simulink model "HarnessModel_MotorDrive"  (R2025a)
settings: Solver=VariableStepAuto  StartTime=0.0  StopTime=0.2  MaxStep=1/2e-6  RelTol=1e-3  AbsTol=1e-3  EnableMultiTasking=on
PreLoadFcn:
  | HarnessSetup_MotorDrive
undefined symbols (not defined in the file or in its folder): foc, PmsmFem, testParams
libraries: nesl_utility x14, ee_lib x12, fl_lib x10, spsFirstOrderFilterLib x4, eePmsmFieldOrientedControl x1
(part 1 of 2)
Description:
  | Three-Phase PMSM Drive
settings Model: Creator=The MathWorks, Inc.  LastModifiedBy=isaacito
settings SolverCC: AutoScaleAbsTol=off  MaxConsecutiveMinStep=2  ZeroCrossAlgorithm=Adaptive  AlgebraicLoopSolver=TrustRegion
settings DataIOCC: LimitDataPoints=on  MaxDataPoints=690000  SaveFormat=Array  InspectSignalLogs=on
settings OptimizationCC: LifeSpan=inf
settings DebuggingCC: UnderspecifiedInitializationDetection=Classic  MergeDetectMultiDrivingBlocksExec=none  MaxConsecutiveZCsMsg=none  IgnoredZcDiagnostic=none  UnconnectedInputMsg=warning  UnconnectedOutputMsg=warning  UnconnectedLineMsg=warning  AllowSymbolicDim=off  PregeneratedLibrarySubsystemCodeDiagnostic=none  SFUnexpectedBacktrackingDiag=warning  SFNoUnconditionalDefaultTransitionDiag=warning  SFExecutionAtInitializationDiag=none  ArithmeticOperatorsInVariantConditions=warning
settings HardwareCC: ProdBitPerPointer=32.0  ProdBitPerSizeT=32.0  ProdBitPerPtrDiffT=32.0  ProdLargestAtomicFloat=None  ProdIntDivRoundTo=Undefined  ProdEndianess=Unspecified  ProdWordSize=32.0  ProdHWDeviceType=32-bit Generic
settings ModelReferenceCC: EnableRefExpFcnMdlSchedulingChecks=on  PropagateSignalLabelsOutOfModel=off
settings SFSimCC: SimUseLocalCustomCode=off  CustomCodeUndefinedFunction=UseInterfaceOnly
settings RTWCC: RTWUseLocalCustomCode=off  GPUComputeCapability=3.5
settings CodeAppCC: StateflowObjectComments=on
settings GRTTargetCC: TargetLangStandard=C89/C90 (ANSI)
settings ConfigComp: CovMetricSettings=dw  CovSaveCumulativeToWorkspaceVar=on  CovSaveSingleToWorkspaceVar=on  CovExternalEMLEnable=off  CovSFcnEnable=off
settings SimscapeCC: SimscapeLogType=local  SimscapeLogName=logsoutssc  SimscapeLogLimitData=off  SimscapeLogDataHistory=1000000.0

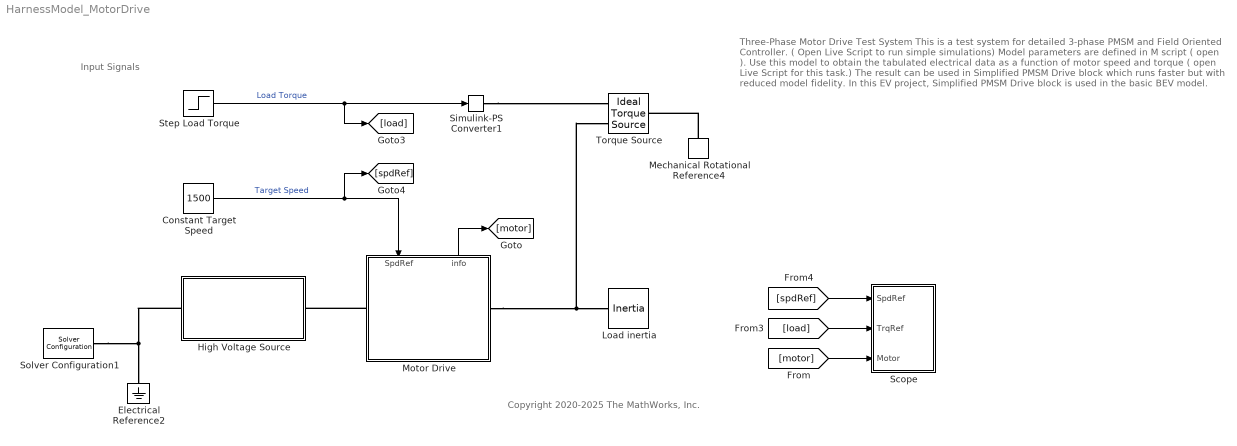
== system HarnessModel_MotorDrive ==
  note: Copyright 2020-2025 The MathWorks, Inc.
  note: Input Signals
  note: Three-Phase Motor Drive Test System
      |
      | This is a test system for detailed 3-phase PMSM and Field Oriented
      | Controller. ( Open Live Script to run simple simulations)
      |
      | Model parameters are defined in M script ( open ).
      |
      | Use this model to obtain the tabulated electrical data as a function of
      | motor speed and torque ( open Live Script for this task.) The result can be
      | used in Simplified PMSM Drive block which runs faster but with reduced
      | model fidelity. In this EV project, Simplified PMSM Drive block is used in
      | the basic BEV model.
  Constant Target Speed : Constant  Value=1500  SampleTime=testParams.controlSampleTime_s
      settings: AttributesFormatString=%<SampleTime>
  Electrical Reference2 : fl_lib/Electrical/Electrical Elements/Electrical Reference
  High Voltage Source : Subsystem
  Load inertia : fl_lib/Mechanical/Rotational Elements/Inertia  inertia=testParams.Load_Inertia_kg_m2 kg*m^2  num_ports=foundation.enum.numPorts2.one  w_specify=on  w_priority=High  w=1500 rpm  w_nominal_specify=off  w_nominal_value=1  w_nominal_unit=rad/s  t_specify=off  t_priority=High  t=0 N*m  t_nominal_specify=off  t_nominal_value=1  t_nominal_unit=N*m
      settings: AttributesFormatString=Initial %<w> %<w_unit>
  Mechanical Rotational Reference4 : fl_lib/Mechanical/Rotational Elements/Mechanical Rotational Reference
  Motor Drive : Subsystem
      settings: PortSchema="{\"entries\":[{\"content\":{\"sides\":[{\"content\":{\"connectorIds\":[\"LConn1\"]},\"type\":\"ConnectorPlacement.EquallySpacedRectSide\",\"uuid\":\"01e463d5-292f-49ad-b53f-26bdaef9861a\"},{\"content\":{\"connectorIds\":[\"RConn1\"],\"side\":\"RIGHT\"},\"type\":\"ConnectorPlacement.EquallySpacedRectSide\",\"uuid\":\"c82e9c8b-ca5a-45cd-a1e1-09f3eb3693bb\"},{\"content\":{\"connectorIds\":[\"In1\",\"Out1\"],\"side\":\"TOP\"},\"type\":\"ConnectorPlacement.EquallySpacedRectSide\",\"uuid\":\"d9b13513-5e9a-4a5c-9a36-dd7bb14f7238\"}]},\"type\":\"ConnectorPlacement.EquallySpacedConnector\",\"uuid\":\"1701c5a8-0236-4c04-8589-5cbcf2c3bfdc\"}],\"packageUris\":[\"http://schema.mathworks.com/mf0/Connector/19700101\"],\"version\":\"1.0\"}"
  Scope : Subsystem
  Simulink-PS Converter1 : nesl_utility/Simulink-PS Converter  PhysicalDomain=network_engine_domain  SubClassName=ps_input  LeftPortType=input  RightPortType=output  PseudoPeriodic=off  Frequencies=[]  NoiseDistribution=none  NoiseParameters=[]  Unit=N*m  AffineConversion=off  FilteringAndDerivatives=provide  SimscapeFilterOrder=1  InputFilterTimeConstant=0.001  UdotUserProvided=0
  Solver Configuration1 : nesl_utility/Solver Configuration  PhysicalDomain=network_engine_domain  SubClassName=solver  LeftPortType=input  RightPortType=generic  Tones=[]  Harmonics=[]  SimulateNoise=off  Profile=off  UseLocalSampling=off  EnableSwitchedLinearOptims=on  FrequencyDomain=off  UseCCode=off  RelTol=0.001  AbsTol=1e-06  MinStep=1e-09  ToWorkspace=off  RevertToSquareIcSolve=off  NumHomotopyIterations=100  PhasorMode=off  PhasorModeNumHarmonics=1  ConsistencySolver=NEWTON_FTOL  IndexReductionMethod=DerivativeReplacement  DoDC=off  ResidualTolerance=1e-9  ConsistencyTolSource=GLOBAL  ConsistencyAbsTol=0.001  ConsistencyRelTol=0.001  ConsistencyTolFactor=0.001  UseLocalSolver=on  LocalSolverChoice=NE_BACKWARD_EULER_ADVANCER  ResolveIndetEquations=on  FunctionEvalNumThread=1  LocalSolverSampleTime=testParams.sampleTime_s  DoFixedCost=on  MaxNonlinIter=5  MaxModeIter=2  ComputeImpulses=off  ImpulseIterations=2  LinearAlgebra=auto  LinearAlgebraNumThread=0  EquationFormulation=NE_TIME_EF  DelaysMemoryBudget=1024  AutomaticFiltering=on  FilteringTimeConstant=0.001  PartitionStorageMethod=AS_NEEDED  PartitionMemoryBudget=1024  PartitionMethod=FAST  MultibodyUseLocalSolver=off  MultibodyLocalSolverChoice=ODE1  MultibodyLocalSolverSampleTime=0.001
      settings: AttributesFormatString=Local solver %<UseLocalSolver>
  Step Load Torque : Step  Time=0.01  After=150  SampleTime=0
      settings: AttributesFormatString=|
      | Initial %<Before>
      | Step to %<After>
  Torque Source : fl_lib/Mechanical/Mechanical Sources/Ideal Torque Source
  wires:
  Step Load Torque/1 -> [load], Simulink-PS Converter1/1  "Load Torque"
  Motor Drive/1(info) -> [motor]
  Constant Target Speed/1 -> [spdRef], Motor Drive/1(SpdRef)  "Target Speed"
  [spdRef] -> Scope/1(SpdRef)
  [load] -> Scope/2(TrqRef)
  [motor] -> Scope/3(Motor)
  connections:
  Motor Drive/RConn1 -- Torque Source/RConn2 -- Load inertia/LConn1
  Simulink-PS Converter1/RConn1 -- Torque Source/RConn1
  Mechanical Rotational Reference4/LConn1 -- Torque Source/LConn1
  Motor Drive/LConn1 -- High Voltage Source/RConn1
  High Voltage Source/LConn1 -- Electrical Reference2/LConn1 -- Solver Configuration1/RConn1

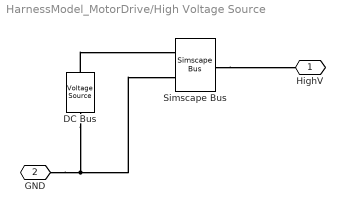
== system HarnessModel_MotorDrive/High Voltage Source ==
  DC Bus : ee_lib/Sources/Voltage Source  dc_voltage=testParams.DC_V V  ac_voltage=0 V  ac_shift=0 deg  ac_frequency=0 Hz  noise_mode=0  PSD=0 V^2/Hz  sample_time=0.001 s  repeatability=1  user_seed=0  auto_seed=2280074224  i_specify=off  i_priority=None  i=0 A  i_nominal_specify=off  i_nominal_value=1  i_nominal_unit=A  v_specify=off  v_priority=None  v=0 V  v_nominal_specify=off  v_nominal_value=1  v_nominal_unit=V
      settings: AttributesFormatString=%<dc_voltage> (%<dc_voltage_unit>)
  Simscape Bus : SimscapeBus  HierarchyStrings=plus;minus
  HighV : PMIOPort  Side=Right
  GND : PMIOPort  Port=2  Side=Left
  connections:
  DC Bus/LConn1 -- Simscape Bus/LConn1
  DC Bus/RConn1 -- GND/RConn1 -- Simscape Bus/LConn2
  Simscape Bus/RConn1 -- HighV/RConn1

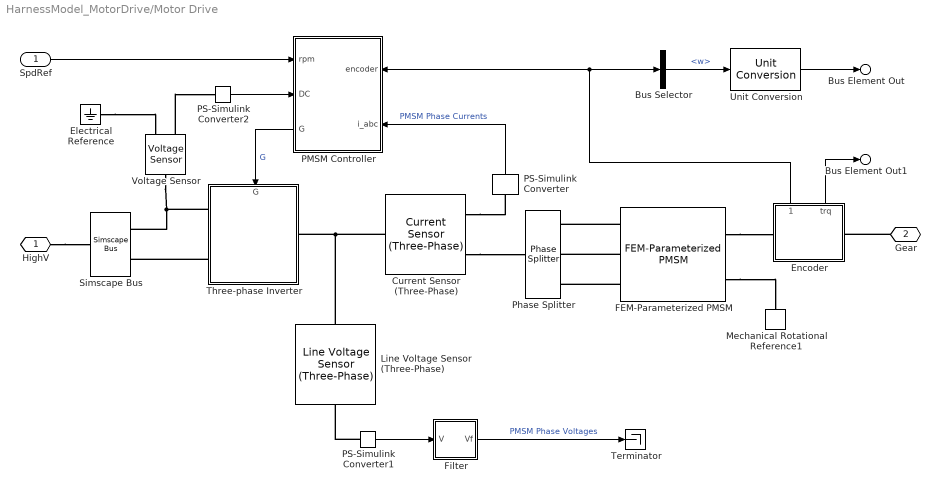
== system HarnessModel_MotorDrive/Motor Drive ==
  SpdRef : Inport  Unit=rpm
  Bus Selector : BusSelector  OutputSignals=w
  Current Sensor (Three-Phase) : ee_lib/Sensors & Transducers/Current Sensor (Three-Phase)
  Electrical Reference : fl_lib/Electrical/Electrical Elements/Electrical Reference
  Encoder : Subsystem
      settings: PortSchema="{\"entries\":[{\"content\":{\"sides\":[{\"content\":{\"connectorIds\":[\"LConn1\"]},\"type\":\"ConnectorPlacement.EquallySpacedRectSide\",\"uuid\":\"cfad22f7-4ca5-4e38-a161-f69c3faf7447\"},{\"content\":{\"connectorIds\":[\"RConn1\"],\"side\":\"RIGHT\"},\"type\":\"ConnectorPlacement.EquallySpacedRectSide\",\"uuid\":\"720e2ecf-f383-4111-97af-41d99d9b093d\"},{\"content\":{\"connectorIds\":[\"Out1\",\"Out2\"],\"side\":\"TOP\"},\"type\":\"ConnectorPlacement.EquallySpacedRectSide\",\"uuid\":\"072894f0-fc0d-4f40-82e8-543eb6144e32\"}]},\"type\":\"ConnectorPlacement.EquallySpacedConnector\",\"uuid\":\"8d289e27-8023-447e-8610-dc73c3ce1339\"}],\"packageUris\":[\"http://schema.mathworks.com/mf0/Connector/19700101\"],\"version\":\"1.0\"}"
  FEM-Parameterized PMSM : ee_lib/Electromechanical/Permanent Magnet/FEM-Parameterized PMSM  parameterization=1  winding_type=ee.enum.statorconnection.wye  iVec=[-2, 0, 2] A  xVec=[0, 20, 40, 60] deg  dfluxdiMatrix=0.0002 * ones(3, 4) Wb/A  dfluxdxMatrix=[0, -.16, .16, 0; 0, -.16, .16, 0; 0, -.16, .16, 0] Wb/rad  calculate_torque_matrix=1  TorqueMatrix=zeros(3, 3, 3, 4) N*m  idVec1=[-200, 0, 200] A  iqVec1=[-200, 0, 200] A  LdMatrix=0.0002 * ones(3, 3) H  LqMatrix=0.0002 * ones(3, 3) H  PmMatrix=0.1 * ones(3, 3) Wb  interp_method=simscape.enum.interpolation.linear  N=6  Rs=PmsmFem.Rs_Ohm Ohm  Ms=0.00002 H  L0=0.00016 H  loss_param=ee.enum.fem_motor.ironLossesExtended.empirical  losses_oc=PmsmFem.openCircuitLossVec_W W  losses_sc=PmsmFem.shortCircuitLossVec_W W  f_losses=PmsmFem.frequencyForLosses_Hz Hz  Isc_losses=PmsmFem.shortCircuitCurrent_A A  Inertia=PmsmFem.rotorInertia_kg_m2 kg*m^2  lam=PmsmFem.rotorDamping_Nm_per_radps N*m/(rad/s)  i_d_specify=on  i_d_priority=High  i_d=PmsmFem.initialDAxisCurrent_A A  i_d_nominal_specify=off  i_d_nominal_value=1  i_d_nominal_unit=A  i_q_specify=on  i_q_priority=High  i_q=PmsmFem.initialQAxisCurrent_A A  i_q_nominal_specify=off  i_q_nominal_value=1  i_q_nominal_unit=A  torque_specify=off  torque_priority=None  torque=0 N*m  torque_nominal_specify=off  torque_nominal_value=1  torque_nominal_unit=N*m  angular_velocity_specify=on  angular_velocity_priority=None  angular_velocity=0 rpm  angular_velocity_nominal_specify=off  angular_velocity_nominal_value=1  angular_velocity_nominal_unit=rpm  angular_position_specify=on  angular_position_priority=High  angular_position=PmsmFem.initialRotorAngle_rad rad  angular_position_nominal_specify=off  angular_position_nominal_value=1  angular_position_nominal_unit=deg  alpha=3.93e-3 1/K  alpha_flux=-0.001 1/K  Tmeas=298.15 K  stator_thermal_mass=100 J/K  stator_initial_temperatures=[298.15, 298.15, 298.15] K  rotor_thermal_mass=200 J/K  rotor_initial_temperature=298.15 K  Rm_percent_rotor=90  Rd_percent_rotor=30  idVec=[-200, 0, 200] A  iqVec=[-200, 0, 200] A  dfluxAdiaMatrix3D=zeros(3, 3, 4) Wb/A  dfluxAdibMatrix3D=zeros(3, 3, 4) Wb/A  dfluxAdicMatrix3D=zeros(3, 3, 4) Wb/A  dfluxAdxMatrix3D=zeros(3, 3, 4) Wb/rad  TorqueMatrix3D=zeros(3, 3, 4) N*m  iaVec=[-200, 0, 200] A  ibVec=[-200, 0, 200] A  icVec=[-200, 0, 200] A  dfluxAdiaMatrix=zeros(3, 3, 3, 4) Wb/A  dfluxAdibMatrix=zeros(3, 3, 3, 4) Wb/A  dfluxAdicMatrix=zeros(3, 3, 3, 4) Wb/A  dfluxAdxMatrix=zeros(3, 3, 3, 4) Wb/rad  param_dq0=ee.enum.fem_motor.fluxTabulationOption.Acartesian  winding_type_dq0=ee.enum.statorconnection.wye  expose_neutral_port=ee.enum.fem_motor.exposeNeutralPort.no  nPolePairs=PmsmFem.NumPolePairs  parks_type=ee.enum.fem_motor.parksType.QleadsD_AphaseToDaxis  idVec2=PmsmFem.idVec_A A  iqVec2=PmsmFem.iqVec_A A  magVec2=[0, 100, 200] A  betaVec2=[-180, -90, 0, 90, 180] deg  xVec2=PmsmFem.angleVec_deg deg  fluxD_dq0=PmsmFem.fluxD_Wb Wb  fluxQ_dq0=PmsmFem.fluxQ_Wb Wb  fluxA_dq0=PmsmFem.flux Wb  Torque_dq0=PmsmFem.torque_Nm N*m  fluxD_IBX=zeros(3, 5, 7) Wb  fluxQ_IBX=zeros(3, 5, 7) Wb  fluxA_IBX=zeros(3, 5, 7) Wb  Torque_IBX=zeros(3, 5, 7) N*m  rotorLossCoeff_k_h_DQ=zeros(3, 3) W/Hz  rotorLossCoeff_k_J_DQ=zeros(3, 3) W/Hz^2  rotorLossCoeff_k_ex_DQ=zeros(3, 3) W/Hz^(3/2)  rotorLossCoeff_k_h_IB=zeros(3, 5) W/Hz  rotorLossCoeff_k_J_IB=zeros(3, 5) W/Hz^2  rotorLossCoeff_k_ex_IB=zeros(3, 5) W/Hz^(3/2)  statorLossCoeff_k_h_DQ=zeros(3, 3) W/Hz  statorLossCoeff_k_J_DQ=zeros(3, 3) W/Hz^2  statorLossCoeff_k_ex_DQ=zeros(3, 3) W/Hz^(3/2)  statorLossCoeff_k_h_IB=zeros(3, 5) W/Hz  statorLossCoeff_k_J_IB=zeros(3, 5) W/Hz^2  statorLossCoeff_k_ex_IB=zeros(3, 5) W/Hz^(3/2)  wVec=[1000, 2000] rpm  rotorLossTable_DQ=zeros(3, 3, 2) W  statorLossTable_DQ=zeros(3, 3, 2) W  rotorLossTable_IB=zeros(3, 5, 2) W  statorLossTable_IB=zeros(3, 5, 2) W  electrical_torque_before_iron_losses_specify=off  electrical_torque_before_iron_losses_priority=None  electrical_torque_before_iron_losses=0 N*m  electrical_torque_before_iron_losses_nominal_specify=off  electrical_torque_before_iron_losses_nominal_value=1  electrical_torque_before_iron_losses_nominal_unit=N*m  Qrotor_specify=off  Qrotor_priority=None  Qrotor=0 J/s  Qrotor_nominal_specify=off  Qrotor_nominal_value=1  Qrotor_nominal_unit=J/s  Qstator_specify=off  Qstator_priority=None  Qstator=0 J/s  Qstator_nominal_specify=off  Qstator_nominal_value=1  Qstator_nominal_unit=J/s
      settings: LogSimulationData=on  InternalSimscapePortConfiguration="{\"Bottom\":[],\"Left\":[{\"id\":\"a\",\"label\":\"a\",\"type\":\"foundation.electrical.electrical\"},{\"id\":\"b\",\"label\":\"b\",\"type\":\"foundation.electrical.electrical\"},{\"id\":\"c\",\"label\":\"c\",\"type\":\"foundation.electrical.electrical\"}],\"Right\":[{\"id\":\"R\",\"label\":\"R\",\"type\":\"foundation.mechanical.rotational.rotational\"},{\"id\":\"C\",\"label\":\"C\",\"type\":\"foundation.mechanical.rotational.rotational\"}],\"Top\":[]}"
  Filter : Subsystem
  Line Voltage Sensor (Three-Phase) : ee_lib/Sensors & Transducers/Line Voltage Sensor (Three-Phase)
  Mechanical Rotational Reference1 : fl_lib/Mechanical/Rotational Elements/Mechanical Rotational Reference
  PMSM Controller : Subsystem
      settings: PortSchema="{\"entries\":[{\"content\":{\"sides\":[{\"content\":{\"connectorIds\":[\"In1\",\"In2\"]},\"type\":\"ConnectorPlacement.EquallySpacedRectSide\",\"uuid\":\"4c32f1a4-bd89-4f05-8eaa-e2dd24abb257\"},{\"content\":{\"connectorIds\":[\"In3\",\"In4\",\"Out1\"],\"side\":\"RIGHT\"},\"type\":\"ConnectorPlacement.EquallySpacedRectSide\",\"uuid\":\"3a536089-b16f-4be7-9641-6e190c11a3d2\"},{\"content\":{\"connectorIds\":[],\"side\":\"TOP\"},\"type\":\"ConnectorPlacement.EquallySpacedRectSide\",\"uuid\":\"a2701a3e-e366-4020-97eb-8b06a1d4835f\"}]},\"type\":\"ConnectorPlacement.EquallySpacedConnector\",\"uuid\":\"63f34eb4-489c-429c-82ff-74daaf150fe3\"}],\"packageUris\":[\"http://schema.mathworks.com/mf0/Connector/19700101\"],\"version\":\"1.0\"}"
  PS-Simulink Converter : nesl_utility/PS-Simulink Converter  PhysicalDomain=network_engine_domain  SubClassName=ps_output  LeftPortType=input  RightPortType=output  PseudoPeriodic=off  Frequencies=[]  VectorFormat=1-D array  Unit=A  AffineConversion=off
  PS-Simulink Converter1 : nesl_utility/PS-Simulink Converter  PhysicalDomain=network_engine_domain  SubClassName=ps_output  LeftPortType=input  RightPortType=output  PseudoPeriodic=off  Frequencies=[]  VectorFormat=1-D array  Unit=V  AffineConversion=off
  PS-Simulink Converter2 : nesl_utility/PS-Simulink Converter  PhysicalDomain=network_engine_domain  SubClassName=ps_output  LeftPortType=input  RightPortType=output  PseudoPeriodic=off  Frequencies=[]  VectorFormat=1-D array  Unit=V  AffineConversion=off
  Phase Splitter : ee_lib/Connectors & References/Phase Splitter
  Simscape Bus : SimscapeBus  HierarchyStrings=plus;minus
  Terminator : Terminator
  Three-phase Inverter : Subsystem
      settings: PortSchema="{\"entries\":[{\"content\":{\"sides\":[{\"content\":{\"connectorIds\":[\"LConn1\",\"LConn2\"]},\"type\":\"ConnectorPlacement.EquallySpacedRectSide\",\"uuid\":\"b77a7b87-9b1e-4a17-b6f6-338fca9d9cfe\"},{\"content\":{\"connectorIds\":[\"RConn1\"],\"side\":\"RIGHT\"},\"type\":\"ConnectorPlacement.EquallySpacedRectSide\",\"uuid\":\"84d00c63-1b9f-4e1b-a87e-6ae3bc20b0e8\"},{\"content\":{\"connectorIds\":[\"In1\"],\"side\":\"TOP\"},\"type\":\"ConnectorPlacement.EquallySpacedRectSide\",\"uuid\":\"34fb6523-0d29-4b30-bf80-8d7a8441c019\"}]},\"type\":\"ConnectorPlacement.EquallySpacedConnector\",\"uuid\":\"8748b1af-e44d-48ba-bbd0-c9117dbbd6f9\"}],\"packageUris\":[\"http://schema.mathworks.com/mf0/Connector/19700101\"],\"version\":\"1.0\"}"
  Unit Conversion : UnitConversion
  Voltage Sensor : fl_lib/Electrical/Electrical Sensors/Voltage Sensor
  HighV : PMIOPort  Side=Left
  Gear : PMIOPort  Port=2  Side=Right
  Bus Element Out : Outport  PortName=info  Element=motorSpd
      settings: AttributesFormatString=%<Unit>
  Bus Element Out1 : Outport  PortName=info  Element=motorTrq
      settings: AttributesFormatString=%<Unit>
  wires:
  PS-Simulink Converter2/1 -> PMSM Controller/4(DC)
  Unit Conversion/1 -> Bus Element Out/1
  PS-Simulink Converter/1 -> PMSM Controller/2(i_abc)  "PMSM Phase Currents"
  Filter/1(Vf) -> Terminator/1  "PMSM Phase Voltages"
  PMSM Controller/1(G) -> Three-phase Inverter/1(G)  "G"
  Encoder/1(encoder) -> PMSM Controller/1(encoder), Bus Selector/1
  PS-Simulink Converter1/1 -> Filter/1(V)
  SpdRef/1 -> PMSM Controller/3(rpm)
  Bus Selector/1 -> Unit Conversion/1  "<w>"
  Encoder/2(trq) -> Bus Element Out1/1
  connections:
  Voltage Sensor/LConn1 -- Three-phase Inverter/LConn1 -- Simscape Bus/LConn1
  Line Voltage Sensor (Three-Phase)/LConn1 -- Three-phase Inverter/RConn1 -- Current Sensor (Three-Phase)/LConn1
  FEM-Parameterized PMSM/RConn2 -- Mechanical Rotational Reference1/LConn1
  FEM-Parameterized PMSM/LConn2 -- Phase Splitter/RConn2
  FEM-Parameterized PMSM/RConn1 -- Encoder/LConn1
  FEM-Parameterized PMSM/LConn3 -- Phase Splitter/RConn3
  Voltage Sensor/RConn1 -- PS-Simulink Converter2/LConn1
  Three-phase Inverter/LConn2 -- Simscape Bus/LConn2
  HighV/RConn1 -- Simscape Bus/RConn1
  Current Sensor (Three-Phase)/RConn1 -- PS-Simulink Converter/LConn1
  Gear/RConn1 -- Encoder/RConn1
  Current Sensor (Three-Phase)/RConn2 -- Phase Splitter/LConn1
  Electrical Reference/LConn1 -- Voltage Sensor/RConn2
  PS-Simulink Converter1/LConn1 -- Line Voltage Sensor (Three-Phase)/RConn1
  FEM-Parameterized PMSM/LConn1 -- Phase Splitter/RConn1

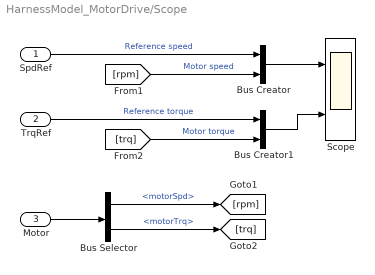
== system HarnessModel_MotorDrive/Scope ==
  SpdRef : Inport
  TrqRef : Inport  Port=2
  Motor : Inport  Port=3
  Bus Creator : BusCreator  Inputs=2
  Bus Creator1 : BusCreator  Inputs=2
  Bus Selector : BusSelector  OutputSignals=motorSpd,motorTrq
  Scope : Scope  NumInputPorts=2
      settings: ActiveDisplayYMinimum=-701.71451342248156  ActiveDisplayYMaximum=-685.71067635737563
  wires:
  Bus Creator1/1 -> Scope/2
  Bus Selector/2 -> [trq]  "<motorTrq>"
  [rpm] -> Bus Creator/2  "Motor speed"
  Bus Selector/1 -> [rpm]  "<motorSpd>"
  [trq] -> Bus Creator1/2  "Motor torque"
  SpdRef/1 -> Bus Creator/1  "Reference speed"
  Bus Creator/1 -> Scope/1
  Motor/1 -> Bus Selector/1
  TrqRef/1 -> Bus Creator1/1  "Reference torque"

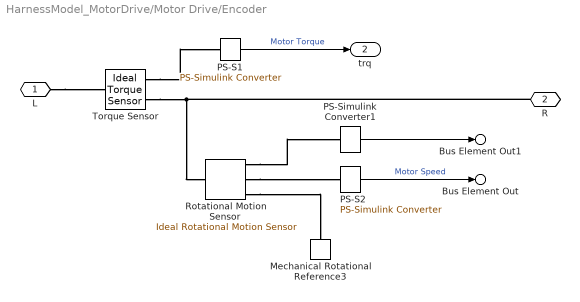
== system HarnessModel_MotorDrive/Motor Drive/Encoder ==
  Mechanical Rotational Reference3 : fl_lib/Mechanical/Rotational Elements/Mechanical Rotational Reference
  PS-S1 : nesl_utility/PS-Simulink Converter  PhysicalDomain=network_engine_domain  SubClassName=ps_output  LeftPortType=input  RightPortType=output  PseudoPeriodic=off  Frequencies=[]  VectorFormat=1-D array  Unit=N*m  AffineConversion=off
  PS-S2 : nesl_utility/PS-Simulink Converter  PhysicalDomain=network_engine_domain  SubClassName=ps_output  LeftPortType=input  RightPortType=output  PseudoPeriodic=off  Frequencies=[]  VectorFormat=1-D array  Unit=rad/s  AffineConversion=off
  PS-Simulink Converter1 : nesl_utility/PS-Simulink Converter  PhysicalDomain=network_engine_domain  SubClassName=ps_output  LeftPortType=input  RightPortType=output  PseudoPeriodic=off  Frequencies=[]  VectorFormat=1-D array  Unit=rad  AffineConversion=off
  Rotational Motion Sensor : fl_lib/Mechanical/Mechanical Sensors/Ideal Rotational Motion Sensor  reference=foundation.enum.MeasurementReference.difference  acceleration_port=false  velocity_port=true  position_port=true  wrap_angle=simscape.enum.onoff.off  offset=0 rad
      settings: LogSimulationData=on
  Torque Sensor : fl_lib/Mechanical/Mechanical Sensors/Ideal Torque Sensor
      settings: LogSimulationData=on
  L : PMIOPort  Side=Left
  R : PMIOPort  Port=2  Side=Right
  Bus Element Out : Outport  PortName=encoder  Element=w
      settings: AttributesFormatString=%<Unit>
  Bus Element Out1 : Outport  PortName=encoder  Element=a
      settings: AttributesFormatString=%<Unit>
  trq : Outport  Port=2
  wires:
  PS-S2/1 -> Bus Element Out/1  "Motor Speed"
  PS-Simulink Converter1/1 -> Bus Element Out1/1
  PS-S1/1 -> trq/1  "Motor Torque"
  connections:
  Rotational Motion Sensor/RConn3 -- PS-Simulink Converter1/LConn1
  Rotational Motion Sensor/RConn2 -- PS-S2/LConn1
  R/RConn1 -- Torque Sensor/RConn1 -- Rotational Motion Sensor/LConn1
  L/RConn1 -- Torque Sensor/LConn1
  Torque Sensor/RConn2 -- PS-S1/LConn1
  Rotational Motion Sensor/RConn1 -- Mechanical Rotational Reference3/LConn1

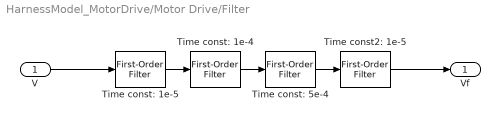
== system HarnessModel_MotorDrive/Motor Drive/Filter ==
  V : Inport
  Time const2: 1e-5 : spsFirstOrderFilterLib/First-Order Filter  FilterType=Lowpass  Tc=1e-5  Ts=0  Initialize=on  Vac_Init=[0, 0, 0]  Vdc_Init=0  PlotResponse=off  FreqRange="[0,  200,  1]"
  Time const: 1e-4 : spsFirstOrderFilterLib/First-Order Filter  FilterType=Lowpass  Tc=1e-4  Ts=0  Initialize=on  Vac_Init=[0, 0, 0]  Vdc_Init=0  PlotResponse=off  FreqRange="[0,  200,  1]"
  Time const: 1e-5 : spsFirstOrderFilterLib/First-Order Filter  FilterType=Lowpass  Tc=1e-5  Ts=0  Initialize=on  Vac_Init=[0, 0, 0]  Vdc_Init=0  PlotResponse=off  FreqRange="[0,  200,  1]"
  Time const: 5e-4 : spsFirstOrderFilterLib/First-Order Filter  FilterType=Lowpass  Tc=5e-4  Ts=0  Initialize=on  Vac_Init=[0, 0, 0]  Vdc_Init=0  PlotResponse=off  FreqRange="[0,  200,  1]"
  Vf : Outport  Unit=V
  wires:
  Time const: 5e-4/1 -> Time const2: 1e-5/1
  Time const: 1e-4/1 -> Time const: 5e-4/1
  Time const: 1e-5/1 -> Time const: 1e-4/1
  V/1 -> Time const: 1e-5/1
  Time const2: 1e-5/1 -> Vf/1

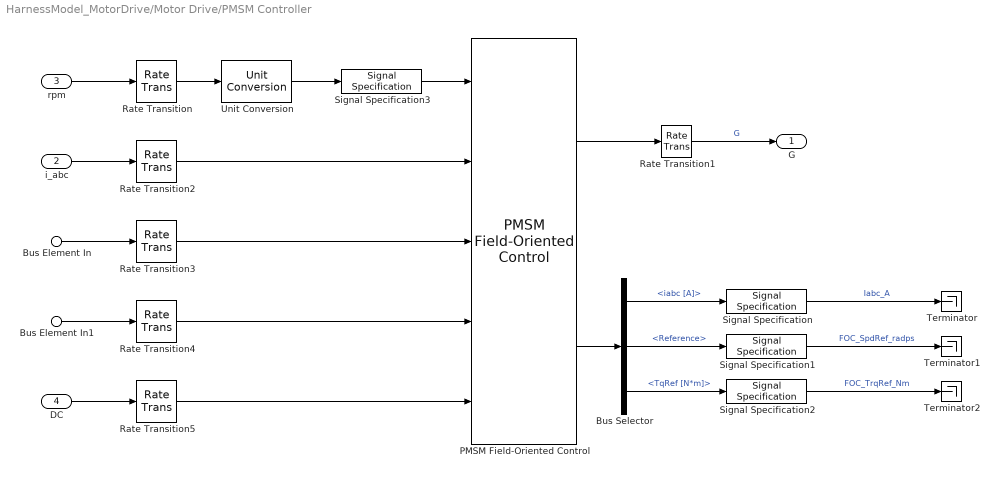
== system HarnessModel_MotorDrive/Motor Drive/PMSM Controller ==
  Bus Element In : Inport  PortName=encoder  Element=w
      settings: AttributesFormatString=%<Unit>
  Bus Element In1 : Inport  PortName=encoder  Element=a
      settings: AttributesFormatString=%<Unit>
  i_abc : Inport  Port=2
  rpm : Inport  Port=3  Unit=rpm
  DC : Inport  Port=4
  Bus Selector : BusSelector  OutputSignals=iabc [A],Reference,TqRef [N*m]
  PMSM Field-Oriented Control : eePmsmFieldOrientedControl/PMSM Field-Oriented Control  winding_type=Wye-wound  CtrlMode=Velocity control  Vnom=foc.nominalDC_V  Pmax=foc.maxPower_W  Tmax=foc.maxTrq_Nm  p=foc.numPolePairs  Vdc_on=foc.DCthresh_V  Ts=foc.sampleTime_s  Tsc=foc.controlSampleTime_s  CtrlType=PI control  Kp_w=25  Ki_w=1000  Kv_w=1  Kaw_w=1  RefType=Zero d-axis control  rpmVec=[0, 1500, 2500, 10000]  TqVec=[-150:10:150]  VdcVec=500  PWMMode=SPWM: sinusoidal PWM  ModFactor=1  idMatrix=zeros(2,3,2)  iqMatrix=zeros(2,3,2)  psim=foc.PM_Wb  Ld=0.00024  Lq=0.00029  Rs=PmsmFem.Rs_Ohm  AxisAlignment=Q-axis  Kp_id=0.7452/2  Ki_id=95.4/2  Kaw_id=0  Kp_iq=2.3993/2  Ki_iq=100  Kaw_iq=930/2  AxisPrio=Q-axis  ActZC=off  ActFF=on  ParamTypeFF=Constant parameters  LdFF=foc.Ld_H  LqFF=foc.Lq_H  psimFF=foc.PM_Wb  idVect=[-200, 0, 200]  iqVect=[-200, 0, 200]  LdMatrix=0.0002 * ones(3, 3)  LqMatrix=0.0002 * ones(3, 3)  psimMatrix=0.04 * ones(3, 3)  CPWMMode=SPWM: sinusoidal PWM  fsw=foc.fsw_Hz
  Rate Transition{,2..4} (4 alike) : RateTransition  OutPortSampleTime=foc.controlSampleTime_s
      settings: AttributesFormatString=%<OutPortSampleTime>
  Rate Transition1 : RateTransition  OutPortSampleTime=foc.sampleTime_s
      settings: AttributesFormatString=%<OutPortSampleTime>
  Rate Transition5 : RateTransition  InitialCondition=foc.initialHighV_V  OutPortSampleTime=foc.controlSampleTime_s
      settings: AttributesFormatString=|
      | %<OutPortSampleTime>
      | Initial Condition: %<InitialCondition>
  Signal Specification : SignalSpecification  Unit=A
  Signal Specification1 : SignalSpecification  Unit=rad/s
  Signal Specification2 : SignalSpecification  Unit=N*m
  Signal Specification3 : SignalSpecification  Unit=rad/s
  Terminator : Terminator
  Terminator1 : Terminator
  Terminator2 : Terminator
  Unit Conversion : UnitConversion
  G : Outport  VectorParamsAs1DForOutWhenUnconnected=off
  wires:
  Bus Selector/1 -> Signal Specification/1  "<iabc [A]>"
  PMSM Field-Oriented Control/2 -> Bus Selector/1
  DC/1 -> Rate Transition5/1
  PMSM Field-Oriented Control/1 -> Rate Transition1/1
  Signal Specification3/1 -> PMSM Field-Oriented Control/1
  Bus Selector/2 -> Signal Specification1/1  "<Reference>"
  Bus Selector/3 -> Signal Specification2/1  "<TqRef [N*m]>"
  Signal Specification/1 -> Terminator/1  "Iabc_A"
  Signal Specification1/1 -> Terminator1/1  "FOC_SpdRef_radps"
  Signal Specification2/1 -> Terminator2/1  "FOC_TrqRef_Nm"
  Unit Conversion/1 -> Signal Specification3/1
  Rate Transition1/1 -> G/1  "G"
  rpm/1 -> Rate Transition/1
  Rate Transition/1 -> Unit Conversion/1
  i_abc/1 -> Rate Transition2/1
  Rate Transition2/1 -> PMSM Field-Oriented Control/2
  Bus Element In/1 -> Rate Transition3/1
  Rate Transition3/1 -> PMSM Field-Oriented Control/3
  Bus Element In1/1 -> Rate Transition4/1
  Rate Transition4/1 -> PMSM Field-Oriented Control/4
  Rate Transition5/1 -> PMSM Field-Oriented Control/5
